simulink library "relay_housing_lib"  (Simulink 8.1)
settings: Solver=ode45  StartTime=0.0  StopTime=10.0  RelTol=1e-3
undefined symbols (not defined in the file): F0, F1, F2, F3, F4, Ts
libraries: relay_modbus_lib x137, rtio_generic_modbus x69, rtlab x10, simulink_extras x10, simulink x6, RMS_lib x4, relay_PLL_lib x3, powerlib_extras x2, relay_ANSI_functions_lib x2, relay_PQSPF_lib x1, powerlib_meascontrol x1, relay_mgc_cmd_lib x1
(part 2 of 3)

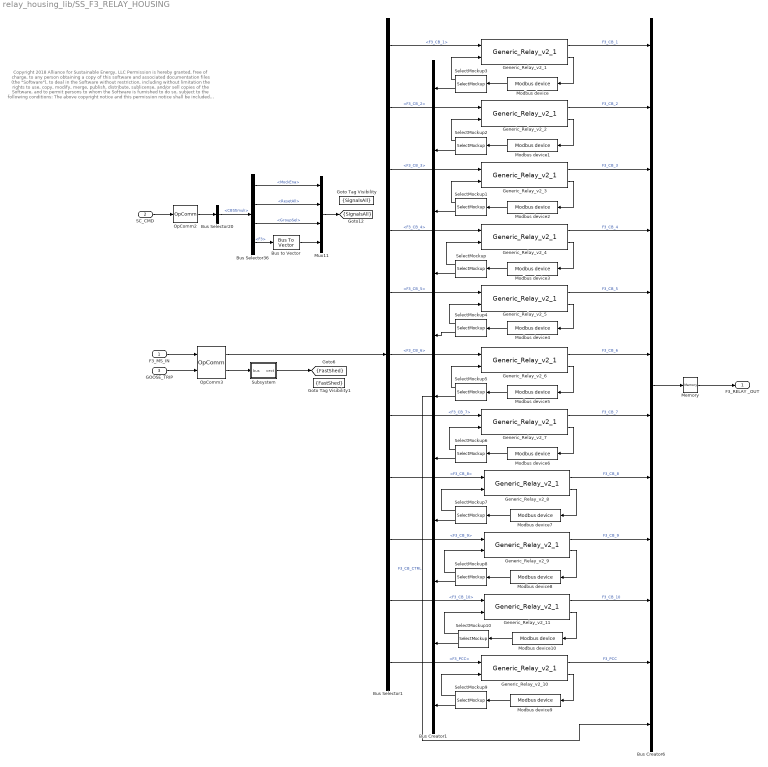
== system relay_housing_lib/SS_F3_RELAY_HOUSING ==
  note: Copyright 2018 Alliance for Sustainable Energy, LLC
      |
      | Permission is hereby granted, free of charge, to any person obtaining a copy of this software
      | and associated documentation files (the "Software"), to deal in the Software without restriction,
      | including without limitation the rights to use, copy, modify, merge, publish, distribute, sublicense,
      | and/or sell copies of the Software, and to permit persons to whom the Software is furnished to do so,
      | subject to the following conditions:
      |
      | The above copyright notice and this permission notice shall be included in all copies or substantial portions of the Software.
      |
      | THE SOFTWARE IS PROVIDED "AS IS", WITHOUT WARRANTY OF ANY KIND, EXPRESS OR IMPLIED, INCLUDING
      | BUT NOT LIMITED TO THE WARRANTIES OF MERCHANTABILITY, FITNESS FOR A PARTICULAR PURPOSE AND
      | NONINFRINGEMENT. IN NO EVENT SHALL THE AUTHORS, THE COPYRIGHT HOLDERS, THE UNITED STATES,
      | THE UNITED STATES DEPARTMENT OF ENERGY, OR ANY OF THEIR EMPLOYEES BE LIABLE FOR ANY CLAIM,
      | DAMAGES OR OTHER LIABILITY, WHETHER IN AN ACTION OF CONTRACT, TORT OR OTHERWISE, ARISING FROM,
      | OUT OF OR IN CONNECTION WITH THE SOFTWARE OR THE USE OR OTHER DEALINGS IN THE SOFTWARE.
  F3_MS_IN : Inport
  SC_CMD : Inport  Port=2
  GOOSE_TRIP : Inport  Port=3
  Bus Creator1 : BusCreator  Inputs=11
  Bus Creator6 : BusCreator  Inputs=12
  Bus Selector1 : BusSelector  OutputSignals=CB_DATA.F3_CB_1,CB_DATA.F3_CB_2,CB_DATA.F3_CB_3,CB_DATA.F3_CB_4,CB_DATA.F3_CB_5,CB_DATA.F3_CB_6,CB_DATA.F3_CB_7,CB_DATA.F3_CB_8,CB_DATA.F3_CB_9,CB_DATA.F3_CB_10,CB_DATA.F3_PCC
  Bus Selector20 : BusSelector  OutputSignals=CBStimuli
  Bus Selector36 : BusSelector  OutputSignals=MockEna,ResetAll,GroupSel,F3
  Bus to Vector : BusToVector
  Generic_Relay_v2_1 : relay_modbus_lib/Generic_Relay_v2_1  Ts=Ts  relay_settings=[F3(1,:)]
  Generic_Relay_v2_10 : relay_modbus_lib/Generic_Relay_v2_1  Ts=Ts  relay_settings=[F0(3,:)]
  Generic_Relay_v2_11 : relay_modbus_lib/Generic_Relay_v2_1  Ts=Ts  relay_settings=[F3(10,:)]
  Generic_Relay_v2_2 : relay_modbus_lib/Generic_Relay_v2_1  Ts=Ts  relay_settings=[F3(2,:)]
  Generic_Relay_v2_3 : relay_modbus_lib/Generic_Relay_v2_1  Ts=Ts  relay_settings=[F3(3,:)]
  Generic_Relay_v2_4 : relay_modbus_lib/Generic_Relay_v2_1  Ts=Ts  relay_settings=[F3(4,:)]
  Generic_Relay_v2_5 : relay_modbus_lib/Generic_Relay_v2_1  Ts=Ts  relay_settings=[F3(5,:)]
  Generic_Relay_v2_6 : relay_modbus_lib/Generic_Relay_v2_1  Ts=Ts  relay_settings=[F3(6,:)]
  Generic_Relay_v2_7 : relay_modbus_lib/Generic_Relay_v2_1  Ts=Ts  relay_settings=[F3(7,:)]
  Generic_Relay_v2_8 : relay_modbus_lib/Generic_Relay_v2_1  Ts=Ts  relay_settings=[F3(8,:)]
  Generic_Relay_v2_9 : relay_modbus_lib/Generic_Relay_v2_1  Ts=Ts  relay_settings=[F3(9,:)]
  Goto Tag Visibility : GotoTagVisibility  GotoTag=SignalsAll
  Goto Tag Visibility1 : GotoTagVisibility  GotoTag=FastShed
  Memory : Memory
  Modbus device : rtio_generic_modbus/Modbus device  conf_name=F3_relay_cfg1.opal  conf_name_mask=F3_relay_cfg1.xls  sample_time=Ts
  Modbus device1 : rtio_generic_modbus/Modbus device  conf_name=F3_relay_cfg2.opal  conf_name_mask=F3_relay_cfg2.xls  sample_time=Ts
  Modbus device10 : rtio_generic_modbus/Modbus device  conf_name=F3_relay_cfg10.opal  conf_name_mask=F3_relay_cfg10.xls  sample_time=Ts
  Modbus device2 : rtio_generic_modbus/Modbus device  conf_name=F3_relay_cfg3.opal  conf_name_mask=F3_relay_cfg3.xls  sample_time=Ts
  Modbus device3 : rtio_generic_modbus/Modbus device  conf_name=F3_relay_cfg4.opal  conf_name_mask=F3_relay_cfg4.xls  sample_time=Ts
  Modbus device4 : rtio_generic_modbus/Modbus device  conf_name=F3_relay_cfg5.opal  conf_name_mask=F3_relay_cfg5.xls  sample_time=Ts
  Modbus device5 : rtio_generic_modbus/Modbus device  conf_name=F3_relay_cfg6.opal  conf_name_mask=F3_relay_cfg6.xls  sample_time=Ts
  Modbus device6 : rtio_generic_modbus/Modbus device  conf_name=F3_relay_cfg7.opal  conf_name_mask=F3_relay_cfg7.xls  sample_time=Ts
  Modbus device7 : rtio_generic_modbus/Modbus device  conf_name=F3_relay_cfg8.opal  conf_name_mask=F3_relay_cfg8.xls  sample_time=Ts
  Modbus device8 : rtio_generic_modbus/Modbus device  conf_name=F3_relay_cfg9.opal  conf_name_mask=F3_relay_cfg9.xls  sample_time=Ts
  Modbus device9 : rtio_generic_modbus/Modbus device  conf_name=F3_relay_cfg_pcc.opal  conf_name_mask=F3_relay_cfg_pcc.xls  sample_time=Ts
  Mux11 : Mux
  OpComm2 : rtlab/OpComm  nbport=1  groupe_acq=1  subsys_rate=0  st=0  Synchronization=on  Interpolation=on  Threshold=1.0  Missed_Data=off  Sim_Time=off  Samples=off  dynSigOut=off  from_console=1  warning_done=off  writeOpCommFile=off  Offset=off
  OpComm3 : rtlab/OpComm  nbport=2  groupe_acq=1  subsys_rate=0  st=0  Synchronization=on  Interpolation=on  Threshold=1.0  Missed_Data=off  Sim_Time=off  Samples=off  dynSigOut=off  from_console=0  warning_done=off  writeOpCommFile=off  Offset=off
  SelectMockup : relay_modbus_lib/SelectMockup  sigID=4  sigN=11
  SelectMockup1 : relay_modbus_lib/SelectMockup  sigID=3  sigN=11
  SelectMockup10 : relay_modbus_lib/SelectMockup  sigID=10  sigN=11
  SelectMockup2 : relay_modbus_lib/SelectMockup  sigID=2  sigN=11
  SelectMockup3 : relay_modbus_lib/SelectMockup  sigID=1  sigN=11
  SelectMockup4 : relay_modbus_lib/SelectMockup  sigID=5  sigN=11
  SelectMockup5 : relay_modbus_lib/SelectMockup  sigID=6  sigN=11
  SelectMockup6 : relay_modbus_lib/SelectMockup  sigID=7  sigN=11
  SelectMockup7 : relay_modbus_lib/SelectMockup  sigID=8  sigN=11
  SelectMockup8 : relay_modbus_lib/SelectMockup  sigID=9  sigN=11
  SelectMockup9 : relay_modbus_lib/SelectMockup  sigID=11  sigN=11
  Subsystem : Subsystem
  F3_RELAY _OUT : Outport
  tag scope: FastShed=scoped, SignalsAll=scoped
  wires:
  Bus Creator1/1 -> Bus Creator6/12  "F3_CB_CTRL"
  SelectMockup9/2 -> Bus Creator1/11
  SelectMockup10/2 -> Bus Creator1/10
  SelectMockup8/2 -> Bus Creator1/9
  SelectMockup7/2 -> Bus Creator1/8
  SelectMockup6/2 -> Bus Creator1/7
  SelectMockup5/2 -> Bus Creator1/6
  SelectMockup4/2 -> Bus Creator1/5
  SelectMockup/2 -> Bus Creator1/4
  SelectMockup1/2 -> Bus Creator1/3
  SelectMockup2/2 -> Bus Creator1/2
  SelectMockup3/2 -> Bus Creator1/1
  Subsystem/1(vect) -> [FastShed]
  OpComm3/2 -> Subsystem/1(bus)
  GOOSE_TRIP/1 -> OpComm3/2
  Bus Selector1/11 -> Generic_Relay_v2_10/1  "<F3_PCC>"
  Modbus device10/1 -> SelectMockup10/1
  SelectMockup10/1 -> Generic_Relay_v2_11/2
  Generic_Relay_v2_11/2 -> Modbus device10/1
  Generic_Relay_v2_11/1 -> Bus Creator6/10  "F3_CB_10"
  Modbus device2/1 -> SelectMockup1/1
  Modbus device/1 -> SelectMockup3/1
  Modbus device1/1 -> SelectMockup2/1
  Modbus device3/1 -> SelectMockup/1
  Modbus device4/1 -> SelectMockup4/1
  Modbus device5/1 -> SelectMockup5/1
  Modbus device6/1 -> SelectMockup6/1
  Modbus device7/1 -> SelectMockup7/1
  Modbus device8/1 -> SelectMockup8/1
  Modbus device9/1 -> SelectMockup9/1
  Mux11/1 -> [SignalsAll]
  Bus Selector36/2 -> Mux11/2  "<ResetAll>"
  Bus Selector36/3 -> Mux11/3  "<GroupSel>"
  Bus to Vector/1 -> Mux11/4
  Bus Selector36/1 -> Mux11/1  "<MockEna>"
  Bus Selector36/4 -> Bus to Vector/1  "<F3>"
  Bus Selector20/1 -> Bus Selector36/1  "<CBStimuli>"
  OpComm2/1 -> Bus Selector20/1
  SC_CMD/1 -> OpComm2/1
  Bus Selector1/10 -> Generic_Relay_v2_11/1  "<F3_CB_10>"
  SelectMockup9/1 -> Generic_Relay_v2_10/2
  Generic_Relay_v2_10/2 -> Modbus device9/1
  Generic_Relay_v2_10/1 -> Bus Creator6/11  "F3_PCC"
  Memory/1 -> F3_RELAY _OUT/1
  Bus Selector1/8 -> Generic_Relay_v2_8/1  "<F3_CB_8>"
  Bus Selector1/9 -> Generic_Relay_v2_9/1  "<F3_CB_9>"
  Generic_Relay_v2_9/1 -> Bus Creator6/9  "F3_CB_9"
  Generic_Relay_v2_8/1 -> Bus Creator6/8  "F3_CB_8"
  SelectMockup8/1 -> Generic_Relay_v2_9/2
  Generic_Relay_v2_9/2 -> Modbus device8/1
  Generic_Relay_v2_8/2 -> Modbus device7/1
  SelectMockup7/1 -> Generic_Relay_v2_8/2
  Bus Creator6/1 -> Memory/1
  Generic_Relay_v2_7/1 -> Bus Creator6/7  "F3_CB_7"
  Generic_Relay_v2_6/1 -> Bus Creator6/6  "F3_CB_6"
  Generic_Relay_v2_5/1 -> Bus Creator6/5  "F3_CB_5"
  Generic_Relay_v2_4/1 -> Bus Creator6/4  "F3_CB_4"
  Generic_Relay_v2_3/1 -> Bus Creator6/3  "F3_CB_3"
  Generic_Relay_v2_2/1 -> Bus Creator6/2  "F3_CB_2"
  Generic_Relay_v2_1/1 -> Bus Creator6/1  "F3_CB_1"
  Bus Selector1/7 -> Generic_Relay_v2_7/1  "<F3_CB_7>"
  Bus Selector1/6 -> Generic_Relay_v2_6/1  "<F3_CB_6>"
  Bus Selector1/5 -> Generic_Relay_v2_5/1  "<F3_CB_5>"
  Bus Selector1/4 -> Generic_Relay_v2_4/1  "<F3_CB_4>"
  Bus Selector1/3 -> Generic_Relay_v2_3/1  "<F3_CB_3>"
  Bus Selector1/2 -> Generic_Relay_v2_2/1  "<F3_CB_2>"
  Bus Selector1/1 -> Generic_Relay_v2_1/1  "<F3_CB_1>"
  F3_MS_IN/1 -> OpComm3/1
  SelectMockup6/1 -> Generic_Relay_v2_7/2
  Generic_Relay_v2_7/2 -> Modbus device6/1
  Generic_Relay_v2_6/2 -> Modbus device5/1
  SelectMockup5/1 -> Generic_Relay_v2_6/2
  SelectMockup4/1 -> Generic_Relay_v2_5/2
  Generic_Relay_v2_5/2 -> Modbus device4/1
  SelectMockup/1 -> Generic_Relay_v2_4/2
  Generic_Relay_v2_4/2 -> Modbus device3/1
  Generic_Relay_v2_3/2 -> Modbus device2/1
  SelectMockup1/1 -> Generic_Relay_v2_3/2
  SelectMockup2/1 -> Generic_Relay_v2_2/2
  Generic_Relay_v2_2/2 -> Modbus device1/1
  SelectMockup3/1 -> Generic_Relay_v2_1/2
  Generic_Relay_v2_1/2 -> Modbus device/1
  OpComm3/1 -> Bus Selector1/1

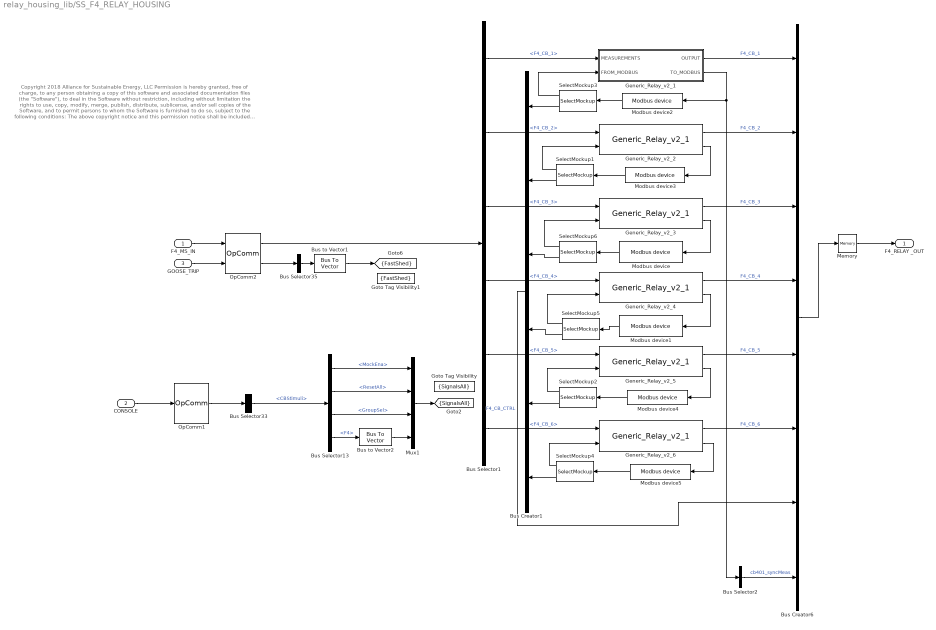
== system relay_housing_lib/SS_F4_RELAY_HOUSING ==
  note: Copyright 2018 Alliance for Sustainable Energy, LLC
      |
      | Permission is hereby granted, free of charge, to any person obtaining a copy of this software
      | and associated documentation files (the "Software"), to deal in the Software without restriction,
      | including without limitation the rights to use, copy, modify, merge, publish, distribute, sublicense,
      | and/or sell copies of the Software, and to permit persons to whom the Software is furnished to do so,
      | subject to the following conditions:
      |
      | The above copyright notice and this permission notice shall be included in all copies or substantial portions of the Software.
      |
      | THE SOFTWARE IS PROVIDED "AS IS", WITHOUT WARRANTY OF ANY KIND, EXPRESS OR IMPLIED, INCLUDING
      | BUT NOT LIMITED TO THE WARRANTIES OF MERCHANTABILITY, FITNESS FOR A PARTICULAR PURPOSE AND
      | NONINFRINGEMENT. IN NO EVENT SHALL THE AUTHORS, THE COPYRIGHT HOLDERS, THE UNITED STATES,
      | THE UNITED STATES DEPARTMENT OF ENERGY, OR ANY OF THEIR EMPLOYEES BE LIABLE FOR ANY CLAIM,
      | DAMAGES OR OTHER LIABILITY, WHETHER IN AN ACTION OF CONTRACT, TORT OR OTHERWISE, ARISING FROM,
      | OUT OF OR IN CONNECTION WITH THE SOFTWARE OR THE USE OR OTHER DEALINGS IN THE SOFTWARE.
  F4_MS_IN : Inport
  CONSOLE : Inport  Port=2
  GOOSE_TRIP : Inport  Port=3
  Bus Creator1 : BusCreator  Inputs=6
  Bus Creator6 : BusCreator  Inputs=8
  Bus Selector1 : BusSelector  OutputSignals=CB_DATA.F4_CB_1,CB_DATA.F4_CB_2,CB_DATA.F4_CB_3,CB_DATA.F4_CB_4,CB_DATA.F4_CB_5,CB_DATA.F4_CB_6
  Bus Selector13 : BusSelector  OutputSignals=MockEna,ResetAll,GroupSel,F4
  Bus Selector2 : BusSelector  OutputSignals=dF,dV,dWt  OutputAsBus=on
  Bus Selector33 : BusSelector  OutputSignals=CBStimuli
  Bus Selector35 : BusSelector  OutputSignals=F4.CB401,F4.CB402,F4.CB403,NA,F4.CB405,F4.CB406  OutputAsBus=on
  Bus to Vector1 : BusToVector
  Bus to Vector2 : BusToVector
  Generic_Relay_v2_1 : Subsystem  AncestorBlock=relay_modbus_lib/Generic_Relay_v2_1  mask(Generic Relay){Ts=Ts, relay_settings=[F4(1,:)]}
      mask prompts: Ts "Sampling Time [Sec]"; relay_settings "Relay Settings"
      mask help:
      | This relay simulates functions: synchronizing or synchronism-check (25), phase instantaneous overcurrent (50P), AC inverse time overcurrent (51P), undervoltage relay (27), and overvoltage relay (59).
      |
      | FEATURES:
      | 1) Receives commands from the microgrid controller via MODBUS/TCP
      | 2) Two groups of interchangeable protection settings
      |     - To be used for grid-tied and islanded protection modes
      | 3) Locked-out only enabled for functions (50P), (51P)
      |     - (27) and (59) pickups will be model inputs for the next revision
      | 4) MODBUS commands expected in the following order:
      |    a) Functions reset (Holding Reg# 2000)
      |    b) Breaker state   (Holding Reg# 2001)
      |    c) Protection mode (Holding Reg# 2002)
      |       - bit = 0; parameter group#1 (default)
      |       - bit = 1; parameter group#2
      |
      | See help or integration packet for further information.
      mask Help:
      | Procedure to reclose a breaker:
      | 1) reset all functions (Holding Reg# 2000)
      | 2) set breaker state (Holding Reg# 2001) to generate a close signal
      | 	- Synch-check (25) will automatically activate
      | 	- bit = 0, trip functions are active
      | 	- bit = 1, trip functions are not active
      | 
      | 
      | 
      | Field format/order for relay settings:
      | 	- Assuming zero delay between group settings changes
      | 
      | 1.  Relay#
      | 2.  Nominal VRMSLL
      | 3.  Max. Slip Voltage [%]
      | 4.  Max. Slip Angle [degree]
      | 5.  Max. Slip Frequency [Hz]
      | 6.  27P and 59P Trip Delay [Sec]
      | 7.  CT Primary
      | 
      | Parameter Group #1
      | 8.  50P Instantaneous overcurrent (IOC) Trip Pickup
      | 9.  50P IOC Trip Delay [sec]
      | 10.  51P Time overcurrent (TOC) Trip Pickup
      | 11.  51P Curve Type
      | 12.  51P TOC Time Dial
      | 13.  27P Trip Pickup [pu]
      | 14.  59P Trip Pickup [pu]
      | 
      | Parameter Group #2
      | 15.  50P IOC Trip Pickup
      | 16.  50P IOC Trip Delay [sec]
      | 17.  51P TOC Trip Pickup
      | 18.  51P Curve Type
      | 19.  51P TOC Time Dial
      | 20.  27P Trip Pickup [pu]
      | 21.  59P Trip Pickup [pu]
      | 
      | Available TCC Characteristics:
      | 	- The degree of inverseness for each curve approximates SEL-751
      | 
      | 51P Curve
      | 1: moderate inverse
      | 2: inverse
      | 3: very inverse
      | 4: extremely inverse
      | 
      | References:
      | [1] IEEE Std. C37.112-1996
      | [2] SEL 751 Instruction manual
      | [3] MIT-LL 2nd Microgrid Controller Symposium - Integration Packet
  Generic_Relay_v2_2 : relay_modbus_lib/Generic_Relay_v2_1  Ts=Ts  relay_settings=[F4(2,:)]
  Generic_Relay_v2_3 : relay_modbus_lib/Generic_Relay_v2_1  Ts=Ts  relay_settings=[F4(3,:)]
  Generic_Relay_v2_4 : relay_modbus_lib/Generic_Relay_v2_1  Ts=Ts  relay_settings=[F4(4,:)]
  Generic_Relay_v2_5 : relay_modbus_lib/Generic_Relay_v2_1  Ts=Ts  relay_settings=[F4(5,:)]
  Generic_Relay_v2_6 : relay_modbus_lib/Generic_Relay_v2_1  Ts=Ts  relay_settings=[F4(6,:)]
  Goto Tag Visibility : GotoTagVisibility  GotoTag=SignalsAll
  Goto Tag Visibility1 : GotoTagVisibility  GotoTag=FastShed
  Memory : Memory
  Modbus device : rtio_generic_modbus/Modbus device  conf_name=F4_relay_cfg3.opal  conf_name_mask=F4_relay_cfg3.xls  sample_time=Ts
  Modbus device1 : rtio_generic_modbus/Modbus device  conf_name=F4_relay_cfg4.opal  conf_name_mask=F4_relay_cfg4.xls  sample_time=Ts
  Modbus device2 : rtio_generic_modbus/Modbus device  conf_name=F4_relay_cfg1.opal  conf_name_mask=F4_relay_cfg1.xls  sample_time=Ts
  Modbus device3 : rtio_generic_modbus/Modbus device  conf_name=F4_relay_cfg2.opal  conf_name_mask=F4_relay_cfg2.xls  sample_time=Ts
  Modbus device4 : rtio_generic_modbus/Modbus device  conf_name=F4_relay_cfg5.opal  conf_name_mask=F4_relay_cfg5.xls  sample_time=Ts
  Modbus device5 : rtio_generic_modbus/Modbus device  conf_name=F4_relay_cfg6.opal  conf_name_mask=F4_relay_cfg6.xls  sample_time=Ts
  Mux1 : Mux
  OpComm1 : rtlab/OpComm  nbport=1  groupe_acq=1  subsys_rate=0  st=0  Synchronization=on  Interpolation=on  Threshold=1.0  Missed_Data=off  Sim_Time=off  Samples=off  dynSigOut=off  from_console=1  warning_done=off  writeOpCommFile=off  Offset=off
  OpComm2 : rtlab/OpComm  nbport=2  groupe_acq=1  subsys_rate=0  st=0  Synchronization=on  Interpolation=on  Threshold=1.0  Missed_Data=off  Sim_Time=off  Samples=off  dynSigOut=off  from_console=0  warning_done=off  writeOpCommFile=off  Offset=off
  SelectMockup1 : relay_modbus_lib/SelectMockup  sigID=2  sigN=6
  SelectMockup2 : relay_modbus_lib/SelectMockup  sigID=5  sigN=6
  SelectMockup3 : relay_modbus_lib/SelectMockup  sigID=1  sigN=6
  SelectMockup4 : relay_modbus_lib/SelectMockup  sigID=6  sigN=6
  SelectMockup5 : relay_modbus_lib/SelectMockup  sigID=4  sigN=6
  SelectMockup6 : relay_modbus_lib/SelectMockup  sigID=3  sigN=6
  F4_RELAY _OUT : Outport
  tag scope: FastShed=scoped, SignalsAll=scoped
  wires:
  Bus Selector2/1 -> Bus Creator6/8  "cb401_syncMeas"
  Generic_Relay_v2_1/2(TO_MODBUS) -> Bus Selector2/1, Modbus device2/1
  Bus Creator1/1 -> Bus Creator6/7  "F4_CB_CTRL"
  SelectMockup4/2 -> Bus Creator1/6
  SelectMockup2/2 -> Bus Creator1/5
  SelectMockup5/2 -> Bus Creator1/4
  SelectMockup6/2 -> Bus Creator1/3
  SelectMockup1/2 -> Bus Creator1/2
  SelectMockup3/2 -> Bus Creator1/1
  Bus to Vector1/1 -> [FastShed]
  Bus Selector35/1 -> Bus to Vector1/1
  OpComm2/2 -> Bus Selector35/1
  GOOSE_TRIP/1 -> OpComm2/2
  OpComm2/1 -> Bus Selector1/1
  F4_MS_IN/1 -> OpComm2/1
  Bus Selector1/1 -> Generic_Relay_v2_1/1(MEASUREMENTS)  "<F4_CB_1>"
  Bus Selector1/2 -> Generic_Relay_v2_2/1  "<F4_CB_2>"
  Bus Selector1/3 -> Generic_Relay_v2_3/1  "<F4_CB_3>"
  Bus Selector1/4 -> Generic_Relay_v2_4/1  "<F4_CB_4>"
  Bus Selector1/5 -> Generic_Relay_v2_5/1  "<F4_CB_5>"
  Bus Selector1/6 -> Generic_Relay_v2_6/1  "<F4_CB_6>"
  Generic_Relay_v2_1/1(OUTPUT) -> Bus Creator6/1  "F4_CB_1"
  Generic_Relay_v2_2/1 -> Bus Creator6/2  "F4_CB_2"
  Generic_Relay_v2_3/1 -> Bus Creator6/3  "F4_CB_3"
  Generic_Relay_v2_4/1 -> Bus Creator6/4  "F4_CB_4"
  Generic_Relay_v2_5/1 -> Bus Creator6/5  "F4_CB_5"
  Generic_Relay_v2_6/1 -> Bus Creator6/6  "F4_CB_6"
  Bus Creator6/1 -> Memory/1
  Memory/1 -> F4_RELAY _OUT/1
  CONSOLE/1 -> OpComm1/1
  OpComm1/1 -> Bus Selector33/1
  Generic_Relay_v2_3/2 -> Modbus device/1
  Generic_Relay_v2_4/2 -> Modbus device1/1
  Modbus device2/1 -> SelectMockup3/1
  SelectMockup3/1 -> Generic_Relay_v2_1/2(FROM_MODBUS)
  Bus Selector33/1 -> Bus Selector13/1  "<CBStimuli>"
  Bus Selector13/4 -> Bus to Vector2/1  "<F4>"
  Bus Selector13/1 -> Mux1/1  "<MockEna>"
  Bus to Vector2/1 -> Mux1/4
  Bus Selector13/3 -> Mux1/3  "<GroupSel>"
  Bus Selector13/2 -> Mux1/2  "<ResetAll>"
  Mux1/1 -> [SignalsAll]
  Generic_Relay_v2_2/2 -> Modbus device3/1
  Modbus device3/1 -> SelectMockup1/1
  SelectMockup1/1 -> Generic_Relay_v2_2/2
  Generic_Relay_v2_5/2 -> Modbus device4/1
  Modbus device4/1 -> SelectMockup2/1
  SelectMockup2/1 -> Generic_Relay_v2_5/2
  Generic_Relay_v2_6/2 -> Modbus device5/1
  Modbus device5/1 -> SelectMockup4/1
  SelectMockup4/1 -> Generic_Relay_v2_6/2
  Modbus device1/1 -> SelectMockup5/1
  SelectMockup5/1 -> Generic_Relay_v2_4/2
  SelectMockup6/1 -> Generic_Relay_v2_3/2
  Modbus device/1 -> SelectMockup6/1

== system relay_housing_lib/SS_F1_RELAY_HOUSING/Subsystem ==
  bus : Inport
  Bus Selector35 : BusSelector  OutputSignals=NA,NA,NA,F1.CB104,NA,NA,F1.CB107,F1.CB108,F1.CB109,F1.CB110,F1.CB111,NA,F1.CB113,F1.CB114,PCC.CB100
  Mux : Mux  Inputs=15
  vect : Outport
  wires:
  Mux/1 -> vect/1
  Bus Selector35/12 -> Mux/12  "<NA>"
  Bus Selector35/1 -> Mux/1  "<NA>"
  Bus Selector35/9 -> Mux/9  "<CB109>"
  Bus Selector35/8 -> Mux/8  "<CB108>"
  Bus Selector35/6 -> Mux/6  "<NA>"
  Bus Selector35/5 -> Mux/5  "<NA>"
  Bus Selector35/13 -> Mux/13  "<CB113>"
  Bus Selector35/10 -> Mux/10  "<CB110>"
  Bus Selector35/14 -> Mux/14  "<CB114>"
  Bus Selector35/11 -> Mux/11  "<CB111>"
  Bus Selector35/15 -> Mux/15  "<CB100>"
  Bus Selector35/4 -> Mux/4  "<CB104>"
  Bus Selector35/2 -> Mux/2  "<NA>"
  Bus Selector35/3 -> Mux/3  "<NA>"
  Bus Selector35/7 -> Mux/7  "<CB107>"
  bus/1 -> Bus Selector35/1

== system relay_housing_lib/SS_F2_RELAY_HOUSING/Subsystem ==
  bus : Inport
  Bus Selector35 : BusSelector  OutputSignals=NA,NA,NA,F2.CB204,NA,F2.CB206,NA,F2.CB208,NA,NA,NA,F2.CB212,F2.CB213,NA,NA,F2.CB216,F2.CB217,F2.CB218,F2.CB219,PCC.CB200
  Mux : Mux  Inputs=20
  vect : Outport
  wires:
  Bus Selector35/1 -> Mux/1  "<NA>"
  Bus Selector35/18 -> Mux/18  "<CB218>"
  Bus Selector35/11 -> Mux/11  "<NA>"
  Bus Selector35/13 -> Mux/13  "<CB213>"
  Bus Selector35/19 -> Mux/19  "<CB219>"
  Bus Selector35/9 -> Mux/9  "<NA>"
  Bus Selector35/7 -> Mux/7  "<NA>"
  Bus Selector35/10 -> Mux/10  "<NA>"
  Bus Selector35/5 -> Mux/5  "<NA>"
  Bus Selector35/8 -> Mux/8  "<CB208>"
  Bus Selector35/6 -> Mux/6  "<CB206>"
  Bus Selector35/15 -> Mux/15  "<NA>"
  Bus Selector35/16 -> Mux/16  "<CB216>"
  Bus Selector35/2 -> Mux/2  "<NA>"
  Bus Selector35/4 -> Mux/4  "<CB204>"
  Bus Selector35/3 -> Mux/3  "<NA>"
  Bus Selector35/20 -> Mux/20  "<CB200>"
  Bus Selector35/14 -> Mux/14  "<NA>"
  Bus Selector35/17 -> Mux/17  "<CB217>"
  Bus Selector35/12 -> Mux/12  "<CB212>"
  Mux/1 -> vect/1
  bus/1 -> Bus Selector35/1

== system relay_housing_lib/SS_F34_RELAY_HOUSING/Subsystem ==
  bus : Inport
  Bus Selector1 : BusSelector  OutputSignals=F4.CB401,F4.CB402,F4.CB403,NA,F4.CB405,F4.CB406  OutputAsBus=on
  Bus Selector35 : BusSelector  OutputSignals=NA,NA,NA,NA,NA,NA,F3.CB307,F3.CB308,F3.CB309,F3.CB310,PCC.CB300
  Bus to Vector1 : BusToVector
  Mux : Mux  Inputs=12
  vect : Outport
  wires:
  Bus to Vector1/1 -> Mux/12
  Bus Selector1/1 -> Bus to Vector1/1
  bus/1 -> Bus Selector35/1, Bus Selector1/1
  Bus Selector35/1 -> Mux/1  "<NA>"
  Bus Selector35/3 -> Mux/3  "<NA>"
  Bus Selector35/11 -> Mux/11  "<CB300>"
  Bus Selector35/4 -> Mux/4  "<NA>"
  Bus Selector35/7 -> Mux/7  "<CB307>"
  Bus Selector35/10 -> Mux/10  "<CB310>"
  Bus Selector35/6 -> Mux/6  "<NA>"
  Bus Selector35/5 -> Mux/5  "<NA>"
  Bus Selector35/2 -> Mux/2  "<NA>"
  Bus Selector35/8 -> Mux/8  "<CB308>"
  Bus Selector35/9 -> Mux/9  "<CB309>"
  Mux/1 -> vect/1

== system relay_housing_lib/SS_F3_RELAY_HOUSING/Subsystem ==
  bus : Inport
  Bus Selector35 : BusSelector  OutputSignals=NA,NA,NA,NA,NA,NA,F3.CB307,F3.CB308,F3.CB309,F3.CB310,PCC.CB300
  Mux : Mux  Inputs=11
  vect : Outport
  wires:
  Bus Selector35/1 -> Mux/1  "<NA>"
  Bus Selector35/3 -> Mux/3  "<NA>"
  Bus Selector35/11 -> Mux/11  "<CB300>"
  Bus Selector35/4 -> Mux/4  "<NA>"
  Bus Selector35/7 -> Mux/7  "<CB307>"
  Bus Selector35/10 -> Mux/10  "<CB310>"
  Bus Selector35/6 -> Mux/6  "<NA>"
  Bus Selector35/5 -> Mux/5  "<NA>"
  Bus Selector35/2 -> Mux/2  "<NA>"
  Bus Selector35/8 -> Mux/8  "<CB308>"
  Bus Selector35/9 -> Mux/9  "<CB309>"
  Mux/1 -> vect/1
  bus/1 -> Bus Selector35/1

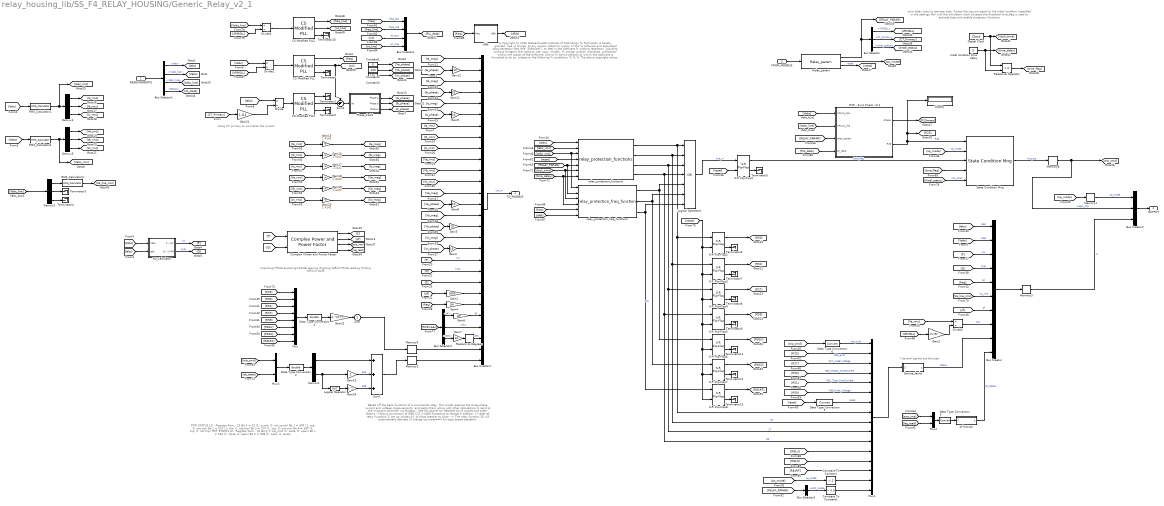
== system relay_housing_lib/SS_F4_RELAY_HOUSING/Generic_Relay_v2_1 ==
  note: % Copyright (c) 2016 Massachusetts Institute of Technology
      | % Permission is hereby granted, free of charge, to any person obtaining a copy of this
      | % software and associated documentation files (the "Software"), to deal in the Software
      | % without restriction, including without limitation the rights to use, copy, modify,
      | % merge, publish, distribute, sublicense, and/or sell copies of the Software, and to
      | % permit persons to whom the Software is furnished to do so, subject to the following
      | % conditions:
      | %
      | %
      | % The above copyright notice and this permission notice shall be included in
      | % all copies or substantial portions of the Software.
      | %
      | % THE SOFTWARE IS PROVIDED "AS IS", WITHOUT WARRANTY OF ANY KIND, EXPRESS OR IMPLIED,
      | % INCLUDING BUT NOT LIMITED TO THE WARRANTIES OF MERCHANTABILITY, FITNESS FOR A
      | % PARTICULAR PURPOSE AND NONINFRINGEMENT. IN NO EVENT SHALL THE AUTHORS OR COPYRIGHT
      | % HOLDERS BE LIABLE FOR ANY CLAIM, DAMAGES OR OTHER LIABILITY, WHETHER IN AN ACTION
      | % OF CONTRACT, TORT OR OTHERWISE, ARISING FROM, OUT OF OR IN CONNECTION WITH THE
      | % SOFTWARE OR THE USE OR OTHER DEALINGS IN THE SOFTWARE.
      | %
      | %
      | %%
  note: Importing=TRUE
      | Exporting=FALSE
      |
      | Lagging (Pushing VARs)=TRUE
      | Leading (Pulling VARs)=FALSE
  note: * several signals are bitwised
  note: Using CT primary to normalize the current.
  note: TRIP STATUS LO - Register Num.: 23
      | Bit 0 = 25  (1: synch, 0: not synch)
      | Bit 1 = 50P (1: trip, 0: not trip)
      | Bit 2 = 51P (1: trip, 0: not trip)
      | Bit 3 = 27P (1: trip, 0: not trip)
      | Bit 4 = 59P (1: trip, 0: not trip)
      |
      | TRIP STATUS HI - Register Num.: 24
      | Bit 0 = trip_cmd  (1: close, 0: open)
      | Bit 1 = 52A (1: close, 0: open)
      | Bit 2 = 52B (1: open, 0: close)
  note: Based off the basic functions of a commercial relay, this model receives
      | the three-phase current and voltage measurements, and packs
      | them along with other calculations to send to the microgrid
      | controller via Modbus
      |
      | - See HIL packet for detailed list of signals and scale factors
      | - Follows convention of IEEE C37.2-2008
      |
      | Procedure to reclose a breaker:
      | 1) reset all relay functions
      | 2) set op_mode==1 to force breaker to close
      |    --> The relay function 25 will automatically activate
      | 3) change op_mode==0 for logic based operation
  note: time delay [sec] to activate logic. Forces the trip_out signal to the initial condition
      | (specified in the settings file) until the simulation clock exceeds the threshold
      |
      | time_flag is used to activate logic and enable protection functions
  MEASUREMENTS : Inport
  FROM_MODBUS : Inport  Port=2
  Bus Creator : BusCreator  Inputs=10
  Bus Creator1 : BusCreator  Inputs=28
  Bus Creator2 : BusCreator  Inputs=3
  Bus Creator3 : BusCreator
  Bus Selector : BusSelector  OutputSignals=VRMSLL,CT_primary,Initial_status
  Bus Selector1 : BusSelector  OutputSignals=Iabc,Vabc_bus,Vabc_line,Status
  Bus Selector2 : BusSelector  OutputSignals=dF,dV,dWt
  Bus Selector3 : BusSelector  OutputSignals=prot_mode
  CS Modified PLL : relay_PLL_lib/CS Modified PLL  Flim=[55 66]  Par_Init=[0 60]  ParK=[ 180 3200 1 ]  Ts=Ts  AGC=off
  CS Modified PLL1 : relay_PLL_lib/CS Modified PLL  Flim=[55 66]  Par_Init=[0 60]  ParK=[ 180 3200 1 ]  Ts=Ts  AGC=off
  CS Modified PLL2 : relay_PLL_lib/CS Modified PLL  Flim=[55 66]  Par_Init=[0 60]  ParK=[ 180 3200 1 ]  Ts=Ts  AGC=off
  Compare To Constant : simulink/Logic and Bit Operations/Compare To Constant  relop=<  const=2  OutDataTypeStr=boolean
  Compare To Constant1 : simulink/Logic and Bit Operations/Compare To Constant  relop=>  const=0.5  OutDataTypeStr=boolean
  Complex Power and Power Factor : relay_PQSPF_lib/Complex Power and Power Factor
  Constant1 : Constant  Value=0
  Constant2 : Constant  Value=-120
  Constant3 : Constant  Value=120
  Data Type Conversion2 : DataTypeConversion  OutDataTypeStr=double
  Data Type Conversion3 : DataTypeConversion
  Data Type Conversion4 : DataTypeConversion  OutDataTypeStr=double
  Data Type Conversion5 : DataTypeConversion
  Data Type Conversion6 : DataTypeConversion
  Demux1 : Demux  Outputs=2
  Demux3 : Demux  Outputs=3
  Demux4 : Demux  Outputs=3
  Demux5 : Demux  Outputs=3
  Digital Clock : DigitalClock  SampleTime=Ts
  Display : Display
  Divide{,1..3} (4 alike) : Product  Inputs=*/
  Gain1 : Gain  Gain=1000
  Gain{3,5,7..9,11..12} (7 alike) : Gain  Gain=10
  Gain13 : Gain  Gain=2
  Gain{15..20} (6 alike) : Gain  Gain=1.4142
  Gain2 : Gain  Gain=1/1.732
  Gain21 : Gain  Gain=1.414
  Gain23 : Gain  Gain=2.^[0:7]
  Gain24 : Gain  Gain=2^2
  Gain4 : Gain  Gain=100
  Gain6 : Gain  Gain=100
  Logical Operator : Logic  Operator=NOT  AllPortsSameDT=off  OutDataTypeStr=boolean
  Logical Operator4 : Logic  Operator=OR  Inputs=7  AllPortsSameDT=off  OutDataTypeStr=boolean
  Memory{1..3,8..9} (5 alike) : Memory
  Mux : Mux  Inputs=8
  Mux1 : Mux  Inputs=16
  Mux2 : Mux  Inputs=2
  Mux3 : Mux  Inputs=2
  PQ_Calculator : Subsystem
  Phase_Calc1 : Subsystem
  R25 - Sync Check v0.1 : Subsystem  AncestorBlock=relay_ANSI_F25_lib/R25 - Sync Check v0.1  mask(Relay synch check){Ts=Ts}
      mask prompts: Ts "Sampling Time [Sec]"
      mask help:
      | This block checks if the the specified conditions for breaker reclosing
      | are met at both terminals of the circuit breaker. This synch check is
      | intended for use in bus-ties, and service lines.
      |
      | The input bus with the relay parameters should be ordered as follows:
      | 1) VRMSLL
      | 2) IOC
      | 3) TOC
      | 4) dV_threshold
      | 5) angle_threshold
      | 6) dF_threshold
  RMS_Calculator1 : RMS_lib/RMS_Calculator  Ts=Ts
  RMS_Calculator2 : RMS_lib/RMS_Calculator  Ts=Ts
  RMS_Calculator3 : RMS_lib/RMS_Calculator  Ts=Ts
  Radians to Degrees : simulink_extras/Transformations/Radians to Degrees
  Relational Operator : RelationalOperator  OutDataTypeStr=boolean
  Relay_param : relay_mgc_cmd_lib/Relay_param  relay_settings=relay_settings
  S-R Flip-Flop{1..8} (8 alike) : simulink_extras/Flip Flops/S-R Flip-Flop  initial_condition=0
  State Condition Mng : relay_tripOutMng_lib/State Condition Mng
  Sum : Sum  Inputs=+
  Sum1 : Sum  Inputs=+++
  Sum2 : Sum  Inputs=-+|
  Terminator{,1..13} (14 alike) : Terminator
  bitwise_faults : Subsystem
  dfdt : Subsystem
  initial condition time delay : Constant  Value=5
  pf bitwise : Subsystem
  relay_protection_freq_functions : relay_ANSI_functions_lib/relay_protection_freq_functions  Ts=Ts
  relay_protection_functions : relay_ANSI_functions_lib/relay_protection_functions  Ts=Ts
  OUTPUT : Outport
  TO_MODBUS : Outport  Port=2
  wires:
  Gain23/1 -> Sum/1
  [R81RF] -> Mux/8
  [R81O] -> Mux/7
  [R81U] -> Mux/6
  Compare To Constant1/1 -> Mux1/16
  Bus Selector3/1 -> Compare To Constant1/1  "<prot_mode>"
  [RELAY_PARAM] -> Bus Selector3/1
  Compare To Constant/1 -> Mux1/15
  [op_mode] -> Compare To Constant/1  "op_mode"
  [R81RF] -> Mux1/14
  [R81O] -> Mux1/13
  [R81U] -> Mux1/12
  relay_protection_freq_functions/2 -> S-R Flip-Flop7/1, Logical Operator4/6
  relay_protection_freq_functions/1 -> Logical Operator4/5, S-R Flip-Flop6/1
  S-R Flip-Flop6/1 -> [R81U]
  S-R Flip-Flop7/1 -> [R81O]
  S-R Flip-Flop8/1 -> [R81RF]
  S-R Flip-Flop8/2 -> Terminator13/1
  S-R Flip-Flop7/2 -> Terminator12/1
  S-R Flip-Flop6/2 -> Terminator11/1
  [reset] -> S-R Flip-Flop2/2, S-R Flip-Flop3/2, S-R Flip-Flop4/2, S-R Flip-Flop5/2, S-R Flip-Flop6/2, S-R Flip-Flop7/2, S-R Flip-Flop8/2
  relay_protection_freq_functions/3 -> Logical Operator4/7, S-R Flip-Flop8/1  "51"
  [dfdt] -> relay_protection_freq_functions/6
  [freq] -> relay_protection_freq_functions/5
  dfdt/1(dfdt) -> [dfdt]
  [freq] -> dfdt/1(freq)
  [wt_line] -> Bus Creator3/4  "wt_line"
  [wt] -> Bus Creator3/3  "wt_bus"
  [freq_line] -> Bus Creator3/2  "freq_line"
  [freq] -> Bus Creator3/1  "freq_bus"
  Bus Creator3/1 -> [PLL_data]
  [PLL_data] -> R25 - Sync Check v0.1/4(pll_data)
  CS Modified PLL2/3 -> Terminator10/1
  CS Modified PLL2/2 -> [wt_line]
  CS Modified PLL2/1 -> [freq_line]
  Divide3/1 -> CS Modified PLL2/1
  [VRMSLL] -> Divide3/2
  [Vabc_line] -> Divide3/1
  Radians to Degrees/1 -> Bus Creator1/26  "dWt"
  Gain7/1 -> Radians to Degrees/1
  Gain6/1 -> Bus Creator1/24  "dF"
  Bus Selector2/3 -> Gain7/1  "<dWt>"
  Bus Selector2/1 -> Gain6/1  "<dF>"
  Bus Selector2/2 -> Bus Creator1/25  "<dV>"
  [R25meas] -> Bus Selector2/1
  R25 - Sync Check v0.1/1(dMeas) -> [R25meas]
  relay_protection_functions/1 -> Logical Operator4/1, S-R Flip-Flop2/1, Mux1/8
  [S] -> Bus Creator1/21
  [Q] -> Bus Creator1/20  "kvar"
  [P] -> Bus Creator1/19  "kw"
  Sum2/1 -> Phase_Calc1/1(wt)
  S-R Flip-Flop2/1 -> [R50]
  S-R Flip-Flop3/1 -> [R51]
  S-R Flip-Flop4/1 -> [R27]
  S-R Flip-Flop5/1 -> [R59]
  S-R Flip-Flop5/2 -> Terminator9/1
  S-R Flip-Flop4/2 -> Terminator8/1
  S-R Flip-Flop3/2 -> Terminator7/1
  S-R Flip-Flop2/2 -> Terminator6/1
  RMS_Calculator3/1 -> [Va_line_rms]
  [Vabc_line] -> Demux3/1
  Relational Operator/1 -> [time_flag]
  Demux3/3 -> Terminator4/1
  Demux3/2 -> Terminator3/1
  Demux3/1 -> RMS_Calculator3/1
  Gain2/1 -> Divide2/2
  Logical Operator/1 -> Gain24/1
  [Initial_status] -> State Condition Mng/5  "init_cond"
  Bus Selector/3 -> [Initial_status]  "<Initial_status>"
  [time_delay] -> relay_protection_freq_functions/4, relay_protection_functions/7
  [clock_time] -> relay_protection_freq_functions/3, relay_protection_functions/6
  Relay_param/3 -> [reset]  "reset"
  initial condition time delay/1 -> [time_delay], Relational Operator/2
  [time_flag] -> State Condition Mng/4
  Digital Clock/1 -> [clock_time], Relational Operator/1
  Gain21/1 -> Divide/2
  Relay_param/2 -> [op_mode]
  [Va_rms] -> Divide2/1
  [VRMSLL] -> Gain2/1
  [VRMSLL] -> Divide1/2
  Divide1/1 -> CS Modified PLL/1
  [Vabc] -> Divide1/1
  Bus Selector/1 -> [VRMSLL]  "<VRMSLL>"
  [RELAY_PARAM] -> R25 - Sync Check v0.1/3(relay_param)
  [RELAY_PARAM] -> relay_protection_freq_functions/2, relay_protection_functions/5
  [Iabc] -> relay_protection_functions/1
  [Vabc_rms] -> relay_protection_freq_functions/1, relay_protection_functions/3
  [Iabc_rms] -> relay_protection_functions/2
  [reset] -> relay_protection_functions/4
  Relay_param/1 -> Bus Selector/1, [RELAY_PARAM]
  Bus Selector/2 -> [CT_Primary]  "<CT_primary>"
  Data Type Conversion3/1 -> pf bitwise/1(S)
  Memory3/1 -> Bus Creator2/3  "m"
  [lag_lead] -> Mux2/2
  [exp_imp] -> Mux2/1
  pf bitwise/1(s) -> Bus Creator/10  "pf_states"
  Mux2/1 -> Data Type Conversion3/1
  Complex Power and Power Factor/4 -> [lag_lead]
  Complex Power and Power Factor/3 -> [exp_imp]
  Complex Power and Power Factor/2 -> [pf]
  Complex Power and Power Factor/1 -> [S]
  [Q] -> Complex Power and Power Factor/2
  [P] -> Complex Power and Power Factor/1
  Bus Creator2/1 -> OUTPUT/1
  Memory1/1 -> Bus Creator2/1  "op_mode"
  Bus Creator/1 -> Memory3/1
  MEASUREMENTS/1 -> Bus Selector1/1
  Bus Selector1/3 -> [Vabc_line]  "<Vabc_line>"
  Bus Selector1/2 -> [Vabc]  "<Vabc_bus>"
  Bus Selector1/1 -> [Iabc]  "<Iabc>"
  [Vabc_line] -> R25 - Sync Check v0.1/2(VPKLN_line)
  Data Type Conversion6/1 -> Mux1/1  "trip_cmd"
  Data Type Conversion5/1 -> Mux1/7  "reset"
  [R59] -> Mux1/6  "R59_Over_Voltage"
  [R51] -> Mux1/5  "R51_Time_OverCurrent"
  [R50] -> Mux1/4  "R50_Instant_OverCurrent"
  [R27] -> Mux1/3  "R27_Under Voltage"
  [R25] -> Mux1/2  "R25_Sync"
  [trip_cmd] -> Data Type Conversion6/1
  [reset] -> Data Type Conversion5/1
  bitwise_faults/1(s) -> Bus Creator/9  "status"
  Mux1/1 -> bitwise_faults/1(S)
  relay_protection_functions/4 -> Logical Operator4/4, S-R Flip-Flop5/1, Mux1/11  "59"
  relay_protection_functions/3 -> Logical Operator4/3, S-R Flip-Flop4/1, Mux1/10  "27"
  Divide2/1 -> Bus Creator/8  "Vpu"
  Gain15/1 -> [Ia_mag]
  Gain16/1 -> [Ib_mag]
  Gain17/1 -> [Ic_mag]
  Gain18/1 -> [Va_mag]
  Gain19/1 -> [Vb_mag]
  Gain20/1 -> [Vc_mag]
  [Vc_rms] -> Gain20/1
  [Vb_rms] -> Gain19/1
  [Va_rms] -> Gain18/1
  [Ic_rms] -> Gain17/1
  [Ib_rms] -> Gain16/1
  [Ia_rms] -> Gain15/1
  [Vabc] -> R25 - Sync Check v0.1/1(VPKLN_bus)
  Gain4/1 -> Bus Creator1/23
  Gain1/1 -> Bus Creator1/22
  Gain3/1 -> Bus Creator1/18
  [Vc_mag] -> Bus Creator1/17
  Gain5/1 -> Bus Creator1/16
  [Vb_mag] -> Bus Creator1/15
  Gain8/1 -> Bus Creator1/14
  [Va_mag] -> Bus Creator1/13
  [Vc_rms] -> Bus Creator1/12
  [Vb_rms] -> Bus Creator1/11
  [Va_rms] -> Bus Creator1/10
  [Ic_rms] -> Bus Creator1/9
  [Ib_rms] -> Bus Creator1/8
  [Ia_rms] -> Bus Creator1/7
  Gain9/1 -> Bus Creator1/6
  [Ic_mag] -> Bus Creator1/5
  Gain11/1 -> Bus Creator1/4
  [Ib_mag] -> Bus Creator1/3
  Gain12/1 -> Bus Creator1/2
  [Ia_mag] -> Bus Creator1/1
  [pf] -> Bus Creator/7  "pf"
  [Va_line_rms] -> Bus Creator/6  "Va_rms"
  [freq] -> Bus Creator/5  "Hz"
  CS Modified PLL/3 -> Terminator/1
  CS Modified PLL1/3 -> Terminator2/1
  CS Modified PLL1/1 -> Terminator1/1
  CS Modified PLL/2 -> Sum2/1, [wt]
  CS Modified PLL/1 -> [freq]
  CS Modified PLL1/2 -> Sum2/2
  S-R Flip-Flop1/1 -> State Condition Mng/3  "fault_flag"
  [op_mode] -> State Condition Mng/2  "op_mode"
  R25 - Sync Check v0.1/2(R25) -> State Condition Mng/1, [R25], Display/1  "R25"
  Memory8/1 -> Bus Creator2/2, [trip_cmd]  "Logic_trip"
  [op_mode] -> Memory1/1
  Memory2/1 -> Bus Creator1/28
  Memory9/1 -> Bus Creator1/27
  Data Type Conversion4/1 -> Gain23/1
  Mux/1 -> Data Type Conversion4/1
  relay_protection_functions/2 -> Logical Operator4/2, S-R Flip-Flop3/1, Mux1/9  "51"
  Sum/1 -> Memory9/1
  Sum1/1 -> Memory2/1
  [Ia_phase] -> Gain12/1
  [Ib_phase] -> Gain11/1
  [Ic_phase] -> Gain9/1
  [Va_phase] -> Gain8/1
  [Vb_phase] -> Gain5/1
  [Vc_phase] -> Gain3/1
  [CT_Primary] -> Gain21/1
  Divide/1 -> CS Modified PLL1/1
  Phase_Calc1/3(Phase c) -> [Ic_phase]
  Phase_Calc1/2(Phase b) -> [Ib_phase]
  Phase_Calc1/1(Phase a) -> [Ia_phase]
  [Iabc] -> Divide/1
  Constant3/1 -> [Vc_phase]
  Constant2/1 -> [Vb_phase]
  Constant1/1 -> [Va_phase]
  [Q] -> Bus Creator/4  "kvar"
  [P] -> Bus Creator/3  "kw"
  [pf] -> Gain1/1
  [freq] -> Gain4/1
  Bus Creator1/1 -> TO_MODBUS/1  "sm_in"
  FROM_MODBUS/1 -> Relay_param/1
  [Vabc] -> Bus Creator/2  "Vabc"
  [Iabc] -> Bus Creator/1  "Iabc"
  [Vabc] -> PQ_Calculator/1(Vabc)
  [Iabc] -> PQ_Calculator/2(Iabc)
  PQ_Calculator/1(P - kW) -> [P]  "kw"
  PQ_Calculator/2(Q - kVAR) -> [Q]  "kvar"
  [Iabc] -> RMS_Calculator1/1
  [Vabc] -> RMS_Calculator2/1
  RMS_Calculator1/1 -> Demux4/1, [Iabc_rms]
  RMS_Calculator2/1 -> Demux5/1, [Vabc_rms]
  Demux4/3 -> [Ic_rms]
  Demux4/2 -> [Ib_rms]
  Demux4/1 -> [Ia_rms]
  Demux5/1 -> [Va_rms]
  Demux5/2 -> [Vb_rms]
  Demux5/3 -> [Vc_rms]
  State Condition Mng/1 -> Memory8/1  "trip_out"
  Bus Selector1/4 -> [cb_state]  "<Status>"
  [R25] -> Mux/1
  [R50] -> Mux/2
  [R51] -> Mux/3
  [R27] -> Mux/4
  [R59] -> Mux/5
  Mux3/1 -> Data Type Conversion2/1
  Gain13/1 -> Sum1/2  "52A"
  Demux1/1 -> Sum1/1
  Data Type Conversion2/1 -> Demux1/1
  [trip_cmd] -> Mux3/1
  [cb_state] -> Mux3/2
  Gain24/1 -> Sum1/3  "52B"
  Demux1/2 -> Logical Operator/1, Gain13/1
  S-R Flip-Flop1/2 -> Terminator5/1
  [reset] -> S-R Flip-Flop1/2
  Logical Operator4/1 -> S-R Flip-Flop1/1  "trip_in"

== system relay_housing_lib/SS_F4_RELAY_HOUSING/Generic_Relay_v2_1/PQ_Calculator ==
  note: Copyright (c) 2016 Massachusetts Institute of Technology
      | Permission is hereby granted, free of charge, to any person obtaining a copy of this software and associated documentation files (the "Software"), to deal
      | in the Software without restriction, including without limitation the rights to use, copy, modify, merge, publish, distribute, sublicense, and/or sell copies of the
      | Software, and to permit persons to whom the Software is furnished to do so, subject to the following conditions:
      |
      | THE SOFTWARE IS PROVIDED "AS IS", WITHOUT WARRANTY OF ANY KIND, EXPRESS OR IMPLIED, INCLUDING BUT NOT LIMITED TO THE
      | WARRANTIES OF MERCHANTABILITY, FITNESS FOR A PARTICULAR PURPOSE AND NONINFRINGEMENT. IN NO EVENT SHALL THE AUTHORS
      | OR COPYRIGHT HOLDERS BE LIABLE FOR ANY CLAIM, DAMAGES OR OTHER LIABILITY, WHETHER IN AN ACTION OF CONTRACT, TORT OR
      | OTHERWISE, ARISING FROM, OUT OF OR IN CONNECTION WITH THE SOFTWARE OR THE USE OR OTHER DEALINGS IN THE SOFTWARE
  Vabc : Inport
  Iabc : Inport  Port=2
  3-phase  Instantaneous  Active & Reactive Power : powerlib_extras/Measurements/3-phase  Instantaneous  Active & Reactive Power
  Demux : Demux  Outputs=2
  Discrete  Mean value2 : powerlib_extras/Discrete Measurements/Discrete  Mean value  Freq=60  Vinit=0  Ts=Ts
  Gain10 : Gain  Gain=1/1000
  P - kW : Outport
  Q - kVAR : Outport  Port=2
  wires:
  Gain10/1 -> Demux/1
  3-phase  Instantaneous  Active & Reactive Power/1 -> Discrete  Mean value2/1
  Discrete  Mean value2/1 -> Gain10/1
  Vabc/1 -> 3-phase  Instantaneous  Active & Reactive Power/1
  Iabc/1 -> 3-phase  Instantaneous  Active & Reactive Power/2
  Demux/1 -> P - kW/1  "kw"
  Demux/2 -> Q - kVAR/1  "kvar"

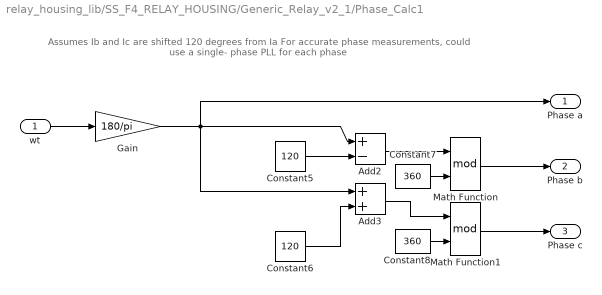
== system relay_housing_lib/SS_F4_RELAY_HOUSING/Generic_Relay_v2_1/Phase_Calc1 ==
  note: Assumes Ib and Ic are shifted 120 degrees from Ia
      | For accurate phase measurements, could use a single-
      | phase PLL for each phase
  wt : Inport
  Add2 : Sum  Inputs=+-
  Add3 : Sum
  Constant5 : Constant  Value=120
  Constant6 : Constant  Value=120
  Constant7 : Constant  Value=360
  Constant8 : Constant  Value=360
  Gain : Gain  Gain=180/pi
  Math Function : Math  Operator=mod  SaturateOnIntegerOverflow=on
  Math Function1 : Math  Operator=mod  SaturateOnIntegerOverflow=on
  Phase a : Outport
  Phase b : Outport  Port=2
  Phase c : Outport  Port=3
  wires:
  Constant5/1 -> Add2/2
  Constant6/1 -> Add3/2
  wt/1 -> Gain/1
  Constant7/1 -> Math Function/2
  Add2/1 -> Math Function/1
  Add3/1 -> Math Function1/1
  Constant8/1 -> Math Function1/2
  Math Function/1 -> Phase b/1
  Math Function1/1 -> Phase c/1
  Gain/1 -> Add3/1, Phase a/1, Add2/1

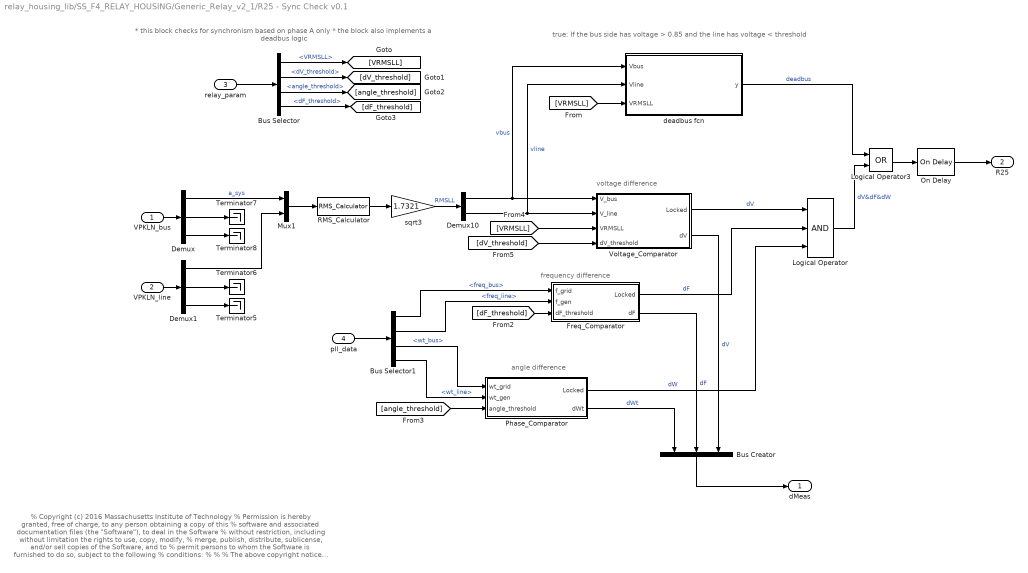
== system relay_housing_lib/SS_F4_RELAY_HOUSING/Generic_Relay_v2_1/R25 - Sync Check v0.1 ==
  note: % Copyright (c) 2016 Massachusetts Institute of Technology
      | % Permission is hereby granted, free of charge, to any person obtaining a copy of this
      | % software and associated documentation files (the "Software"), to deal in the Software
      | % without restriction, including without limitation the rights to use, copy, modify,
      | % merge, publish, distribute, sublicense, and/or sell copies of the Software, and to
      | % permit persons to whom the Software is furnished to do so, subject to the following
      | % conditions:
      | %
      | %
      | % The above copyright notice and this permission notice shall be included in
      | % all copies or substantial portions of the Software.
      | %
      | % THE SOFTWARE IS PROVIDED "AS IS", WITHOUT WARRANTY OF ANY KIND, EXPRESS OR IMPLIED,
      | % INCLUDING BUT NOT LIMITED TO THE WARRANTIES OF MERCHANTABILITY, FITNESS FOR A
      | % PARTICULAR PURPOSE AND NONINFRINGEMENT. IN NO EVENT SHALL THE AUTHORS OR COPYRIGHT
      | % HOLDERS BE LIABLE FOR ANY CLAIM, DAMAGES OR OTHER LIABILITY, WHETHER IN AN ACTION
      | % OF CONTRACT, TORT OR OTHERWISE, ARISING FROM, OUT OF OR IN CONNECTION WITH THE
      | % SOFTWARE OR THE USE OR OTHER DEALINGS IN THE SOFTWARE.
      | %
      | %
      | %%
  note: true: If the bus side has voltage > 0.85 and the line has voltage < threshold
  note: voltage difference
  note: frequency difference
  note: angle difference
  note: * this block checks for synchronism based on phase A only
      | * the block also implements a deadbus logic
  VPKLN_bus : Inport
  VPKLN_line : Inport  Port=2
  relay_param : Inport  Port=3
  pll_data : Inport  Port=4
  Bus Creator : BusCreator  Inputs=3
  Bus Selector : BusSelector  OutputSignals=VRMSLL,dV_threshold,angle_threshold,dF_threshold
  Bus Selector1 : BusSelector  OutputSignals=freq_bus,freq_line,wt_bus,wt_line
  Demux : Demux  Outputs=3
  Demux1 : Demux  Outputs=3
  Demux10 : Demux  Outputs=2
  Freq_Comparator : Subsystem
  Logical Operator : Logic  Inputs=3  AllPortsSameDT=off  OutDataTypeStr=boolean
  Logical Operator3 : Logic  Operator=OR  AllPortsSameDT=off  OutDataTypeStr=boolean
  Mux1 : Mux  Inputs=2
  On Delay : powerlib_meascontrol/Logic/On Delay  DelayType=On delay  delay=0.05  ic=0  Ts=Ts
  Phase_Comparator : Subsystem
  RMS_Calculator : RMS_lib/RMS_Calculator  Ts=Ts
  Terminator{5..8} (4 alike) : Terminator
  Voltage_Comparator : Subsystem
  deadbus fcn : MATLAB Function  TreatAsAtomicUnit=on
  sqrt3 : Gain  Gain=1.7321
  dMeas : Outport
  R25 : Outport  Port=2
  wires:
  On Delay/1 -> R25/1
  Logical Operator3/1 -> On Delay/1
  pll_data/1 -> Bus Selector1/1
  Logical Operator/1 -> Logical Operator3/2  "dV&dF&dW"
  deadbus fcn/1(y) -> Logical Operator3/1  "deadbus"
  VPKLN_line/1 -> Demux1/1
  VPKLN_bus/1 -> Demux/1
  Demux/3 -> Terminator8/1
  Demux/2 -> Terminator7/1
  Demux1/3 -> Terminator5/1
  Demux1/2 -> Terminator6/1
  Demux1/1 -> Mux1/2
  Demux/1 -> Mux1/1  "a_sys"
  Demux10/1 -> Voltage_Comparator/1(V_bus), deadbus fcn/1(Vbus)  "vbus"
  Bus Selector1/1 -> Freq_Comparator/1(f_grid)  "<freq_bus>"
  Bus Selector1/2 -> Freq_Comparator/2(f_gen)  "<freq_line>"
  Bus Selector1/3 -> Phase_Comparator/1(wt_grid)  "<wt_bus>"
  Bus Selector1/4 -> Phase_Comparator/2(wt_gen)  "<wt_line>"
  Demux10/2 -> Voltage_Comparator/2(V_line), deadbus fcn/2(Vline)  "vline"
  Voltage_Comparator/1(Locked) -> Logical Operator/1  "dV"
  Freq_Comparator/1(Locked) -> Logical Operator/2  "dF"
  Phase_Comparator/1(Locked) -> Logical Operator/3  "dW"
  RMS_Calculator/1 -> sqrt3/1
  Mux1/1 -> RMS_Calculator/1
  sqrt3/1 -> Demux10/1  "RMSLL"
  [VRMSLL] -> deadbus fcn/3(VRMSLL)
  relay_param/1 -> Bus Selector/1
  Bus Selector/1 -> [VRMSLL]  "<VRMSLL>"
  Bus Selector/2 -> [dV_threshold]  "<dV_threshold>"
  Bus Selector/3 -> [angle_threshold]  "<angle_threshold>"
  Bus Selector/4 -> [dF_threshold]  "<dF_threshold>"
  [dF_threshold] -> Freq_Comparator/3(dF_threshold)
  [angle_threshold] -> Phase_Comparator/3(angle_threshold)
  [VRMSLL] -> Voltage_Comparator/3(VRMSLL)
  [dV_threshold] -> Voltage_Comparator/4(dV_threshold)
  Voltage_Comparator/2(dV) -> Bus Creator/3  "dV"
  Freq_Comparator/2(dF) -> Bus Creator/2  "dF"
  Phase_Comparator/2(dWt) -> Bus Creator/1  "dWt"
  Bus Creator/1 -> dMeas/1

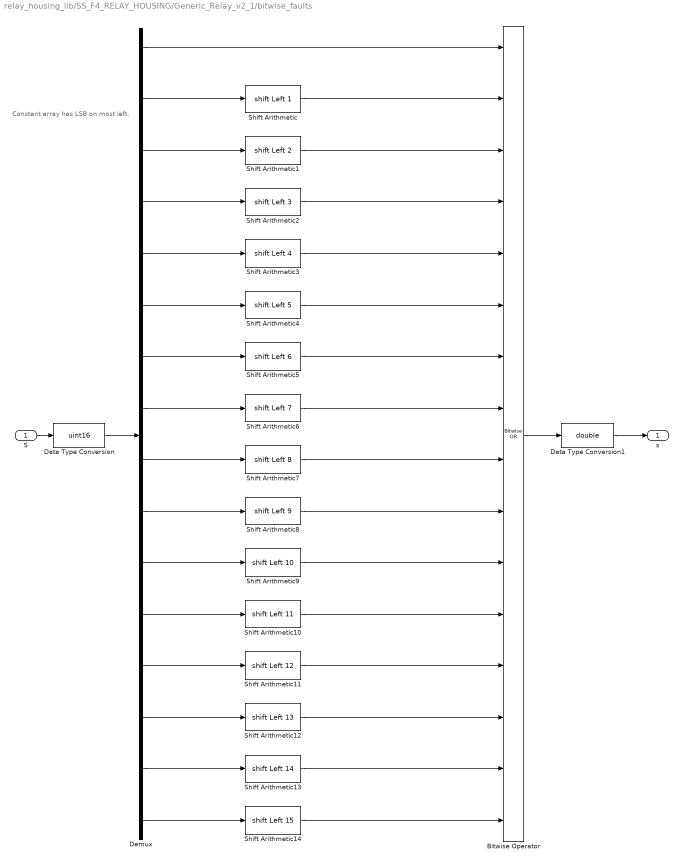
== system relay_housing_lib/SS_F4_RELAY_HOUSING/Generic_Relay_v2_1/bitwise_faults ==
  note: Constant array has LSB on most left.
  S : Inport
  Bitwise Operator : simulink/Logic and Bit Operations/Bitwise Operator  logicop=OR  UseBitMask=off  NumInputPorts=16  BitMask=bin2dec('11011001')  BitMaskRealWorld=Stored Integer
  Data Type Conversion : DataTypeConversion  OutDataTypeStr=uint16
  Data Type Conversion1 : DataTypeConversion  OutDataTypeStr=double
  Demux : Demux  Outputs=16
  Shift Arithmetic : ArithShift  BitShiftNumber=1  BitShiftDirection=Left
  Shift Arithmetic1 : ArithShift  BitShiftNumber=2  BitShiftDirection=Left
  Shift Arithmetic10 : ArithShift  BitShiftNumber=11  BitShiftDirection=Left
  Shift Arithmetic11 : ArithShift  BitShiftNumber=12  BitShiftDirection=Left
  Shift Arithmetic12 : ArithShift  BitShiftNumber=13  BitShiftDirection=Left
  Shift Arithmetic13 : ArithShift  BitShiftNumber=14  BitShiftDirection=Left
  Shift Arithmetic14 : ArithShift  BitShiftNumber=15  BitShiftDirection=Left
  Shift Arithmetic2 : ArithShift  BitShiftNumber=3  BitShiftDirection=Left
  Shift Arithmetic3 : ArithShift  BitShiftNumber=4  BitShiftDirection=Left
  Shift Arithmetic4 : ArithShift  BitShiftNumber=5  BitShiftDirection=Left
  Shift Arithmetic5 : ArithShift  BitShiftNumber=6  BitShiftDirection=Left
  Shift Arithmetic6 : ArithShift  BitShiftNumber=7  BitShiftDirection=Left
  Shift Arithmetic7 : ArithShift  BitShiftNumber=8  BitShiftDirection=Left
  Shift Arithmetic8 : ArithShift  BitShiftNumber=9  BitShiftDirection=Left
  Shift Arithmetic9 : ArithShift  BitShiftNumber=10  BitShiftDirection=Left
  s : Outport
  wires:
  Shift Arithmetic14/1 -> Bitwise Operator/16
  Shift Arithmetic13/1 -> Bitwise Operator/15
  Shift Arithmetic12/1 -> Bitwise Operator/14
  Shift Arithmetic11/1 -> Bitwise Operator/13
  Shift Arithmetic10/1 -> Bitwise Operator/12
  Demux/16 -> Shift Arithmetic14/1
  Demux/15 -> Shift Arithmetic13/1
  Demux/14 -> Shift Arithmetic12/1
  Demux/13 -> Shift Arithmetic11/1
  Demux/12 -> Shift Arithmetic10/1
  Demux/11 -> Shift Arithmetic9/1
  Demux/10 -> Shift Arithmetic8/1
  Demux/9 -> Shift Arithmetic7/1
  Demux/8 -> Shift Arithmetic6/1
  Shift Arithmetic7/1 -> Bitwise Operator/9
  Shift Arithmetic8/1 -> Bitwise Operator/10
  Shift Arithmetic6/1 -> Bitwise Operator/8
  Shift Arithmetic9/1 -> Bitwise Operator/11
  Shift Arithmetic5/1 -> Bitwise Operator/7
  Shift Arithmetic4/1 -> Bitwise Operator/6
  Shift Arithmetic3/1 -> Bitwise Operator/5
  Shift Arithmetic2/1 -> Bitwise Operator/4
  Shift Arithmetic1/1 -> Bitwise Operator/3
  Shift Arithmetic/1 -> Bitwise Operator/2
  Demux/7 -> Shift Arithmetic5/1
  Demux/6 -> Shift Arithmetic4/1
  Demux/5 -> Shift Arithmetic3/1
  Demux/4 -> Shift Arithmetic2/1
  Demux/3 -> Shift Arithmetic1/1
  Demux/2 -> Shift Arithmetic/1
  Demux/1 -> Bitwise Operator/1
  Data Type Conversion1/1 -> s/1
  Bitwise Operator/1 -> Data Type Conversion1/1
  S/1 -> Data Type Conversion/1
  Data Type Conversion/1 -> Demux/1

== system relay_housing_lib/SS_F4_RELAY_HOUSING/Generic_Relay_v2_1/dfdt ==
  note: Hz
  note: Hz/s
  freq : Inport
  Delay1 : Delay  DelayLength=3/60/(Ts)  UseCircularBuffer=on
  Gain : Gain  Gain=60/3
  Sum3 : Sum  Inputs=|-+
  dfdt : Outport
  wires:
  Gain/1 -> dfdt/1  "dfdt"
  Delay1/1 -> Sum3/1
  Sum3/1 -> Gain/1  "df"
  freq/1 -> Delay1/1, Sum3/2

== system relay_housing_lib/SS_F4_RELAY_HOUSING/Generic_Relay_v2_1/pf bitwise ==
  note: Constant array has LSB on most left.
  S : Inport
  Bitwise Operator : simulink/Logic and Bit Operations/Bitwise Operator  logicop=OR  UseBitMask=off  NumInputPorts=2  BitMask=bin2dec('11011001')  BitMaskRealWorld=Stored Integer
  Data Type Conversion : DataTypeConversion  OutDataTypeStr=uint16
  Data Type Conversion1 : DataTypeConversion  OutDataTypeStr=double
  Demux : Demux  Outputs=2
  Shift Arithmetic : ArithShift  BitShiftNumber=1  BitShiftDirection=Left
  s : Outport
  wires:
  Data Type Conversion/1 -> Demux/1
  S/1 -> Data Type Conversion/1
  Bitwise Operator/1 -> Data Type Conversion1/1
  Data Type Conversion1/1 -> s/1
  Demux/1 -> Bitwise Operator/1
  Demux/2 -> Shift Arithmetic/1
  Shift Arithmetic/1 -> Bitwise Operator/2

== system relay_housing_lib/SS_F4_RELAY_HOUSING/Generic_Relay_v2_1/R25 - Sync Check v0.1/Freq_Comparator ==
  note: This block compares the frequency at the circuit breaker terminals
      | * if the difference is less than threshold dF_threshold, then outputs 1
  f_grid : Inport
  f_gen : Inport  Port=2
  dF_threshold : Inport  Port=3
  Fcn2 : Fcn  Expr=abs(u(2)-u(1)) <= u(3)
  Mux1 : Mux  Inputs=3
  Sum : Sum  Inputs=+-
  Locked : Outport
  dF : Outport  Port=2
  wires:
  Mux1/1 -> Fcn2/1
  Fcn2/1 -> Locked/1
  dF_threshold/1 -> Mux1/3
  f_gen/1 -> Sum/1, Mux1/2
  f_grid/1 -> Sum/2, Mux1/1
  Sum/1 -> dF/1
